simulink model "p5"  (R2020b)
settings: Solver=VariableStepAuto  StartTime=0.0  StopTime=35  RelTol=1e-3
undefined symbols (not defined in the file): A, A1, B, B1, C, C1, K, K1, KDelay, L
settings Model: Creator=Julian  LastModifiedBy=Julian

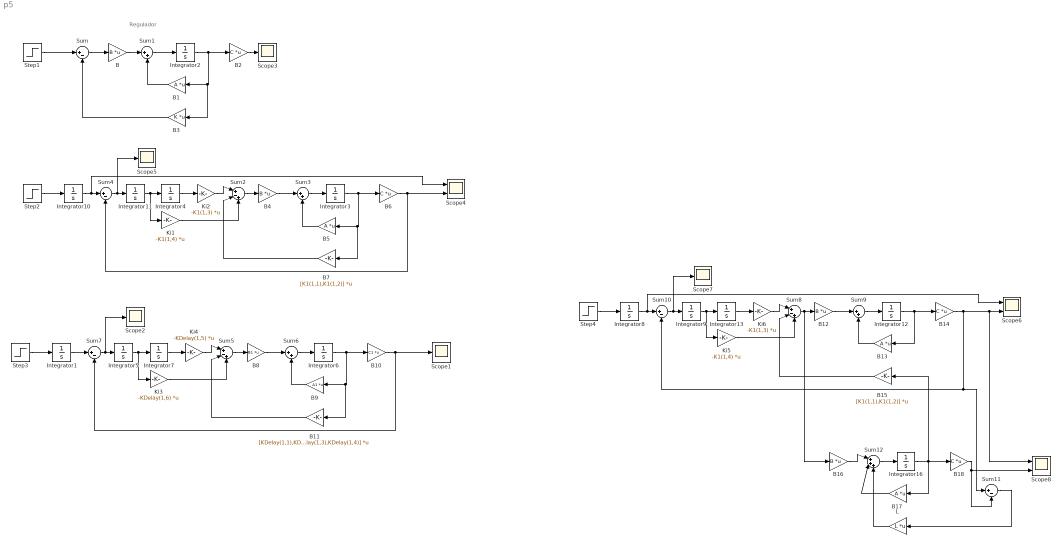
== system p5 ==
  note: Regulador
  B{,4,12,16} (4 alike) : Gain  Gain=B  Multiplication=Matrix(K*u)
  B{1,5,13,17} (4 alike) : Gain  Gain=A  Multiplication=Matrix(K*u)
  B10 : Gain  Gain=C1  Multiplication=Matrix(K*u)
  B11 : Gain  Gain=[KDelay(1,1),KDelay(1,2),KDelay(1,3),KDelay(1,4)]  Multiplication=Matrix(K*u)
  B{2,6,14,18} (4 alike) : Gain  Gain=C  Multiplication=Matrix(K*u)
  B15 : Gain  Gain=[K1(1,1),K1(1,2)]  Multiplication=Matrix(K*u)
  B3 : Gain  Gain=K  Multiplication=Matrix(K*u)
  B7 : Gain  Gain=[K1(1,1),K1(1,2)]  Multiplication=Matrix(K*u)
  B8 : Gain  Gain=B1  Multiplication=Matrix(K*u)
  B9 : Gain  Gain=A1  Multiplication=Matrix(K*u)
  Integrator{1..13,16} (14 alike) : Integrator
  Ki1 : Gain  Gain=-K1(1,4)  Multiplication=Matrix(K*u)
  Ki2 : Gain  Gain=-K1(1,3)  Multiplication=Matrix(K*u)
  Ki3 : Gain  Gain=-KDelay(1,6)  Multiplication=Matrix(K*u)
  Ki4 : Gain  Gain=-KDelay(1,5)  Multiplication=Matrix(K*u)
  Ki5 : Gain  Gain=-K1(1,4)  Multiplication=Matrix(K*u)
  Ki6 : Gain  Gain=-K1(1,3)  Multiplication=Matrix(K*u)
  L : Gain  Gain=L  Multiplication=Matrix(K*u)
  Scope{1..3,5,7} (5 alike) : Scope
  Scope4 : Scope  NumInputPorts=2
  Scope6 : Scope  NumInputPorts=2
  Scope8 : Scope  NumInputPorts=2
  Step{1..4} (4 alike) : Step  Time=0  SampleTime=0
  Sum{,4,7,10..11} (5 alike) : Sum  Inputs=|+-
  Sum{1,3,6,9} (4 alike) : Sum  Inputs=|++
  Sum12 : Sum  Inputs=|+++
  Sum2 : Sum  Inputs=|+-+
  Sum5 : Sum  Inputs=|+-+
  Sum8 : Sum  Inputs=|+-+
  wires:
  B3/1 -> Sum/2
  Sum1/1 -> Integrator2/1
  B2/1 -> Scope3/1
  B1/1 -> Sum1/2
  Step1/1 -> Sum/1
  Sum/1 -> B/1
  B/1 -> Sum1/1
  Integrator2/1 -> B2/1, B3/1, B1/1
  Sum2/1 -> B4/1
  Step2/1 -> Integrator10/1
  Integrator10/1 -> Scope4/1, Sum4/1
  Sum4/1 -> Scope5/1, Integrator11/1
  Sum3/1 -> Integrator3/1
  B5/1 -> Sum3/2
  B7/1 -> Sum2/2
  B4/1 -> Sum3/1
  Ki1/1 -> Sum2/3
  Ki2/1 -> Sum2/1
  Integrator11/1 -> Ki1/1, Integrator4/1
  Integrator4/1 -> Ki2/1
  B6/1 -> Sum4/2, Scope4/2
  Integrator3/1 -> B6/1, B7/1, B5/1
  Integrator6/1 -> B10/1, B11/1, B9/1
  Integrator5/1 -> Ki3/1, Integrator7/1
  B10/1 -> Scope1/1, Sum7/2
  Integrator7/1 -> Ki4/1
  Sum7/1 -> Scope2/1, Integrator5/1
  Ki4/1 -> Sum5/1
  Ki3/1 -> Sum5/3
  B9/1 -> Sum6/2
  B8/1 -> Sum6/1
  Sum5/1 -> B8/1
  B11/1 -> Sum5/2
  Integrator1/1 -> Sum7/1
  Step3/1 -> Integrator1/1
  Sum6/1 -> Integrator6/1
  Integrator12/1 -> B14/1, B13/1
  Integrator9/1 -> Ki5/1, Integrator13/1
  B14/1 -> Sum11/1, Sum10/2, Scope8/1, Scope6/2
  Integrator13/1 -> Ki6/1
  Sum10/1 -> Scope7/1, Integrator9/1
  Ki6/1 -> Sum8/1
  Ki5/1 -> Sum8/3
  B13/1 -> Sum9/2
  B12/1 -> Sum9/1
  B15/1 -> Sum8/2
  Integrator8/1 -> Scope6/1, Sum10/1
  Step4/1 -> Integrator8/1
  Sum9/1 -> Integrator12/1
  Integrator16/1 -> B15/1, B18/1, B17/1
  B17/1 -> Sum12/2
  B16/1 -> Sum12/1
  Sum8/1 -> B16/1, B12/1
  L/1 -> Sum12/3
  Sum12/1 -> Integrator16/1
  B18/1 -> Scope8/2, Sum11/2
  Sum11/1 -> L/1
